simulink model "Electromagnet_Mass_Gravity_System"  (R2025a)
settings: Solver=VariableStepAuto  StartTime=0.0  StopTime=T_sim  RelTol=1e-3  AbsTol=1e-3
PreLoadFcn:
  | init_simscape_simulation
InitFcn:
  | init_simscape_simulation
values from neighbouring files (symbols this model uses):
  Mass = 10    [init_simscape_simulation.m]
  T_sim = 0.2    [init_simscape_simulation.m]
libraries: fl_lib x11, nesl_utility x5
settings Model: Creator=Meng Lingbing  LastModifiedBy=CelestialAurora
settings SolverCC: AutoScaleAbsTol=off  AlgebraicLoopSolver=TrustRegion  MaxZcPerStep=1.0
settings DebuggingCC: UnconnectedInputMsg=warning  UnconnectedOutputMsg=warning  UnconnectedLineMsg=warning  SymbolicDimsDataTypeCodeGenerationDiagnostic=none
settings ModelReferenceCC: EnableRefExpFcnMdlSchedulingChecks=on
settings SFSimCC: CustomCodeUndefinedFunction=UseInterfaceOnly
settings RTWCC: GPUComputeCapability=3.5  DLArmComputeVersion=19.05
settings SimscapeCC: SimscapeLogType=all  SimscapeLogSimulationStatistics=on  SimscapeLogDataHistory=10000.0

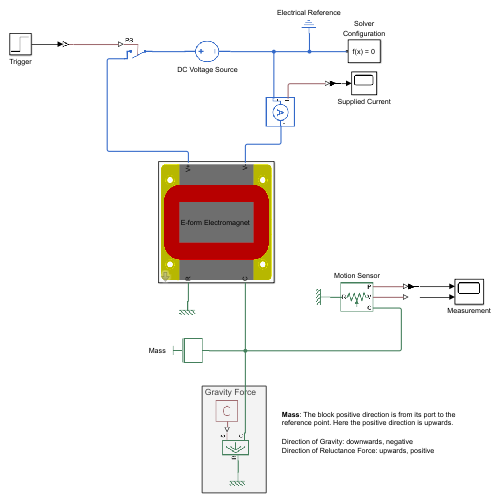
[thumbnail: Simulink's stored preview of the top-level diagram]
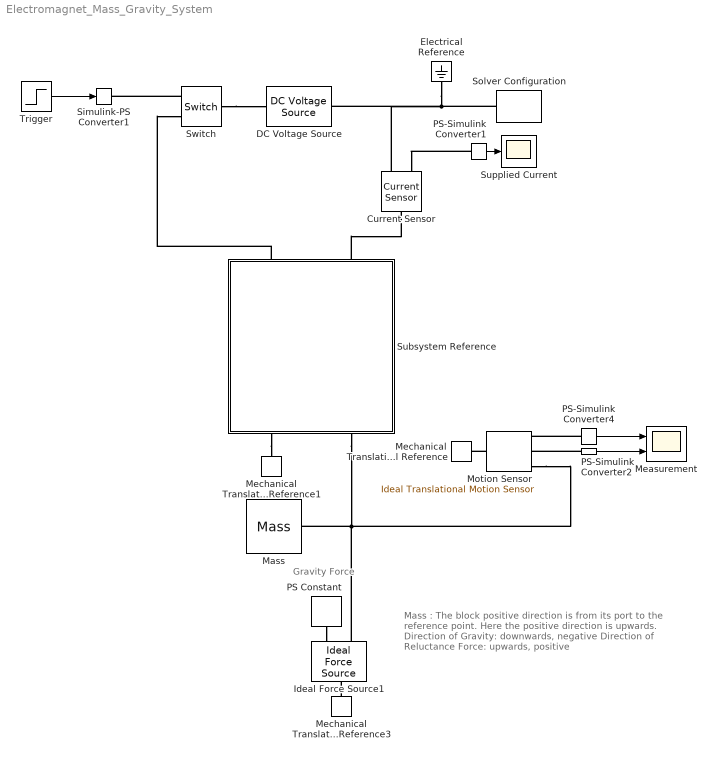
== system Electromagnet_Mass_Gravity_System ==
  note: Mass : The block positive direction is from its port to the reference point. Here the positive direction is upwards.
      |
      | Direction of Gravity: downwards, negative
      | Direction of Reluctance Force: upwards, positive
  note: Gravity Force
  Current Sensor : fl_lib/Electrical/Electrical Sensors/Current Sensor
  DC Voltage Source : fl_lib/Electrical/Electrical Sources/DC Voltage Source  v0=48 V
  Electrical Reference : fl_lib/Electrical/Electrical Elements/Electrical Reference
  Ideal Force Source1 : fl_lib/Mechanical/Mechanical Sources/Ideal Force Source
  Mass : fl_lib/Mechanical/Translational Elements/Mass  mass=Mass kg  num_ports=foundation.enum.numPorts2.one  v_specify=off  v_priority=High  v=0 m/s  v_nominal_specify=off  v_nominal_value=1  v_nominal_unit=m/s  f_specify=off  f_priority=None  f=0 N  f_nominal_specify=on  f_nominal_value=700  f_nominal_unit=N
  Measurement : Scope  NumInputPorts=2
      settings: Title=Velocity  ActiveDisplayYMinimum=-35.897080818152638  ActiveDisplayYMaximum=24.792596731060662
  Mechanical Translational Reference : fl_lib/Mechanical/Translational Elements/Mechanical Translational Reference
  Mechanical Translational Reference1 : fl_lib/Mechanical/Translational Elements/Mechanical Translational Reference
  Mechanical Translational Reference3 : fl_lib/Mechanical/Translational Elements/Mechanical Translational Reference
  Motion Sensor : fl_lib/Mechanical/Mechanical Sensors/Ideal Translational Motion Sensor  reference=foundation.enum.MeasurementReference.difference  acceleration_port=false  velocity_port=true  position_port=true  offset=airgap_init mm
  PS Constant : fl_lib/Physical Signals/Sources/PS Constant  constant=Mass*9.81 N
  PS-Simulink Converter1 : nesl_utility/PS-Simulink Converter  PhysicalDomain=network_engine_domain  SubClassName=ps_output  LeftPortType=input  RightPortType=output  PseudoPeriodic=off  Frequencies=[]  VectorFormat=inherit  Unit=inherit  AffineConversion=off
  PS-Simulink Converter2 : nesl_utility/PS-Simulink Converter  PhysicalDomain=network_engine_domain  SubClassName=ps_output  LeftPortType=input  RightPortType=output  PseudoPeriodic=off  Frequencies=[]  VectorFormat=inherit  Unit=inherit  AffineConversion=off
  PS-Simulink Converter4 : nesl_utility/PS-Simulink Converter  PhysicalDomain=network_engine_domain  SubClassName=ps_output  LeftPortType=input  RightPortType=output  PseudoPeriodic=off  Frequencies=[]  VectorFormat=inherit  Unit=inherit  AffineConversion=off
  Simulink-PS Converter1 : nesl_utility/Simulink-PS Converter  PhysicalDomain=network_engine_domain  SubClassName=ps_input  LeftPortType=input  RightPortType=output  PseudoPeriodic=off  Frequencies=[]  NoiseDistribution=none  NoiseParameters=[]  Unit=1  AffineConversion=off  FilteringAndDerivatives=provide  SimscapeFilterOrder=1  InputFilterTimeConstant=0.001  UdotUserProvided=0
  Solver Configuration : nesl_utility/Solver Configuration  PhysicalDomain=network_engine_domain  SubClassName=solver  LeftPortType=input  RightPortType=generic  Tones=[]  Harmonics=[]  SimulateNoise=off  Profile=off  UseLocalSampling=off  EnableSwitchedLinearOptims=on  FrequencyDomain=off  UseCCode=off  RelTol=0.001  AbsTol=1e-06  MinStep=1e-09  ToWorkspace=off  RevertToSquareIcSolve=off  NumHomotopyIterations=100  PhasorMode=off  PhasorModeNumHarmonics=1  ConsistencySolver=NEWTON_XTOL_AFTER_FTOL  IndexReductionMethod=DerivativeReplacement  DoDC=off  ResidualTolerance=1e-09  ConsistencyTolSource=GLOBAL  ConsistencyAbsTol=0.001  ConsistencyRelTol=0.001  ConsistencyTolFactor=0.001  UseLocalSolver=off  LocalSolverChoice=NE_BACKWARD_EULER_ADVANCER  ResolveIndetEquations=on  FunctionEvalNumThread=1  LocalSolverSampleTime=0.001  DoFixedCost=off  MaxNonlinIter=3  MaxModeIter=2  ComputeImpulses=off  ImpulseIterations=2  LinearAlgebra=auto  LinearAlgebraNumThread=0  EquationFormulation=NE_TIME_EF  DelaysMemoryBudget=1024  AutomaticFiltering=on  FilteringTimeConstant=0.001  PartitionStorageMethod=AS_NEEDED  PartitionMemoryBudget=1024  PartitionMethod=ROBUST  MultibodyUseLocalSolver=off  MultibodyLocalSolverChoice=ODE1  MultibodyLocalSolverSampleTime=0.001
  Subsystem Reference : Subsystem  ReferencedSubsystem=IntegratedElectromagnet  l_airgap=airgap_init
  Supplied Current : Scope
      settings: ActiveDisplayYMinimum=-27.26193  ActiveDisplayYMaximum=245.35735  DataLoggingVariableName=ScopeData2
  Switch : fl_lib/Electrical/Electrical Elements/Switch  R_closed=0.01 Ohm  G_open=1e-08 1/Ohm  Threshold=0  i_specify=off  i_priority=High  i=0 A  i_nominal_specify=off  i_nominal_value=1  i_nominal_unit=A  v_specify=off  v_priority=High  v=0 V  v_nominal_specify=off  v_nominal_value=1  v_nominal_unit=V
  Trigger : Step  Time=0.25*T_sim  SampleTime=0
  wires:
  PS-Simulink Converter4/1 -> Measurement/1
  PS-Simulink Converter1/1 -> Supplied Current/1
  Trigger/1 -> Simulink-PS Converter1/1
  PS-Simulink Converter2/1 -> Measurement/2
  connections:
  Switch/RConn1 -- Simulink-PS Converter1/RConn1
  Solver Configuration/RConn1 -- Current Sensor/RConn2 -- DC Voltage Source/RConn1 -- Electrical Reference/LConn1
  PS-Simulink Converter4/LConn1 -- Motion Sensor/RConn3
  PS-Simulink Converter1/LConn1 -- Current Sensor/RConn1
  Switch/LConn1 -- DC Voltage Source/LConn1
  Subsystem Reference/LConn1 -- Switch/RConn2
  Subsystem Reference/LConn2 -- Current Sensor/LConn1
  PS Constant/RConn1 -- Ideal Force Source1/RConn1
  PS-Simulink Converter2/LConn1 -- Motion Sensor/RConn2
  Subsystem Reference/RConn1 -- Mechanical Translational Reference1/LConn1
  Mechanical Translational Reference3/LConn1 -- Ideal Force Source1/LConn1
  Ideal Force Source1/RConn2 -- Mass/LConn1 -- Subsystem Reference/RConn2 -- Motion Sensor/RConn1
  Motion Sensor/LConn1 -- Mechanical Translational Reference/LConn1
